simulink model "Robust_performance_controller_block"  (R2023b)
settings: Solver=VariableStepAuto  StartTime=0.0  StopTime=10.0  RelTol=1e-3
settings Model: Creator=sarth  LastModifiedBy=sarth

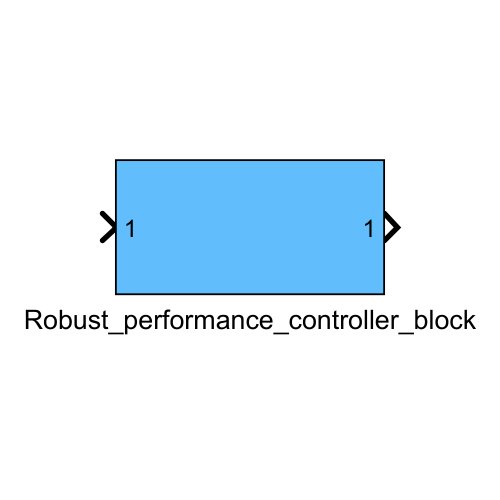
[thumbnail: Simulink's stored preview of the top-level diagram]
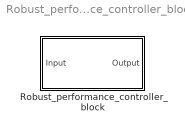
== system Robust_performance_controller_block ==
  Robust_performance_controller_block : Subsystem

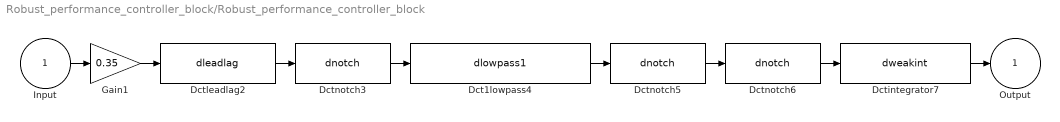
== system Robust_performance_controller_block/Robust_performance_controller_block ==
  Input : Inport
  Dct1lowpass4 : S-Function  FunctionName=dlowpass1  Parameters=f_den, 0.001  SFunctionDeploymentMode=off  EnableBusSupport=off  mask(dctools){f_den=200}
      mask prompts: f_den "Pole [Hz]"
      mask help: This block implements a discrete time 1st order lowpass filter.
      mask Display: disp('DCT 1st order lowpass')
  Dctintegrator7 : S-Function  FunctionName=dweakint  Parameters=f_num, 0.001  SFunctionDeploymentMode=off  EnableBusSupport=off  mask(dctools){f_num=1.5}
      mask prompts: f_num "Zero [Hz]"
      mask help: This block implements a discrete time weak integrator filter.
      mask Display: disp('DCT integrator')
  Dctleadlag2 : S-Function  FunctionName=dleadlag  Parameters=f_num, f_den, 0.001  SFunctionDeploymentMode=off  EnableBusSupport=off  mask(dctools){f_num=2.6, f_den=200}
      mask prompts: f_num "Zero [Hz]"; f_den "Pole [Hz]"
      mask help: This block implements a discrete time leadlag filter.
      mask Display: disp('DCT leadlag')
  Dctnotch3 : S-Function  FunctionName=dnotch  Parameters=f_num, b_num, f_den, b_den, 0.001  SFunctionDeploymentMode=off  EnableBusSupport=off  mask(dctools){f_num=58, b_num=0.0159, f_den=150, b_den=0.3}
      mask prompts: f_num "Zero [Hz]"; b_num "Damping zero [-]"; f_den "Pole [Hz]"; b_den "Damping pole [-]"
      mask help: This block implements a dicrete time 2nd order notch filter.
      mask Display: disp('DCT notch')
  Dctnotch5 : S-Function  FunctionName=dnotch  Parameters=f_num, b_num, f_den, b_den, 0.001  SFunctionDeploymentMode=off  EnableBusSupport=off  mask(dctools){f_num=3, b_num=0.5, f_den=4, b_den=0.05}
      mask prompts: f_num "Zero [Hz]"; b_num "Damping zero [-]"; f_den "Pole [Hz]"; b_den "Damping pole [-]"
      mask help: This block implements a dicrete time 2nd order notch filter.
      mask Display: disp('DCT notch')
  Dctnotch6 : S-Function  FunctionName=dnotch  Parameters=f_num, b_num, f_den, b_den, 0.001  SFunctionDeploymentMode=off  EnableBusSupport=off  mask(dctools){f_num=57, b_num=0.1, f_den=56, b_den=0.3}
      mask prompts: f_num "Zero [Hz]"; b_num "Damping zero [-]"; f_den "Pole [Hz]"; b_den "Damping pole [-]"
      mask help: This block implements a dicrete time 2nd order notch filter.
      mask Display: disp('DCT notch')
  Gain1 : Gain  Gain=0.35
  Output : Outport
  wires:
  Input/1 -> Gain1/1
  Gain1/1 -> Dctleadlag2/1
  Dctleadlag2/1 -> Dctnotch3/1
  Dctnotch3/1 -> Dct1lowpass4/1
  Dct1lowpass4/1 -> Dctnotch5/1
  Dctnotch5/1 -> Dctnotch6/1
  Dctnotch6/1 -> Dctintegrator7/1
  Dctintegrator7/1 -> Output/1
